simulink model "DeltaWingPlantADRC"  (R2020b)
settings: Solver=VariableStepAuto  StartTime=0.0  StopTime=60  MaxStep=0.01  RelTol=1e-3  EnableMultiTasking=on
values from neighbouring files (symbols this model uses):
  B = [0; 1]    [init.m]    (also in init_adrc.m = [0; theta6; 0])
  Ba = Ta*B    [init_adrc.m]
  beta0 = 0.4    [init_adrc.m]
  betap0 = 0    [init_adrc.m]
  gamma = A - L*C    [init_adrc.m]
  gamma_a = I + Ta*gamma    [init_adrc.m]
  kd = 2*wc + theta20    (= 6.29818530718)    [init_adrc.m]
  kp = wc^2+ theta10    (= 9.85160440109)    [init_adrc.m]
  L = [l1; l2; l3]    [init_adrc.m]
  La = Ta*L    [init_adrc.m]
  Ta = 0.04    [init_adrc.m]    (also in init_miac.m = 0.05)
  Tc = 0.1    [init_adrc.m]    (also in init_miac.m = 0.001; init_mrac.m; init_mraclb.m)
  theta10 = -0.018    [init_adrc.m]
  theta20 = 0.015    [init_adrc.m]
  theta6 = 0.5    [init_adrc.m]
libraries: simulink x2
settings Model: Creator=Melkamu A  LastModifiedBy=Melkamu A
settings DataIOCC: LimitDataPoints=on  SaveFormat=Array  SignalLoggingSaveFormat=ModelDataLogs  ReturnWorkspaceOutputs=off
settings OptimizationCC: InitFltsAndDblsToZero=on  LifeSpan=inf
settings DebuggingCC: SaveWithParameterizedLinksMsg=none  UnderspecifiedInitializationDetection=Classic  MergeDetectMultiDrivingBlocksExec=none  SignalResolutionControl=TryResolveAllWithWarning  SolverPrmCheckMsg=warning  MultiTaskDSMMsg=warning  MultiTaskCondExecSysMsg=none  FcnCallInpInsideContextMsg=warning  SFUnexpectedBacktrackingDiag=warning  SFNoUnconditionalDefaultTransitionDiag=warning  SFExecutionAtInitializationDiag=none  ArithmeticOperatorsInVariantConditions=warning
settings HardwareCC: ProdBitPerPointer=32  ProdBitPerSizeT=32  ProdBitPerPtrDiffT=32  ProdLargestAtomicFloat=None  ProdIntDivRoundTo=Undefined  ProdEndianess=Unspecified  ProdWordSize=32  ProdHWDeviceType=32-bit Generic
settings ModelReferenceCC: PropagateSignalLabelsOutOfModel=off
settings CodeAppCC: StateflowObjectComments=on
settings GRTTargetCC: TargetFcnLib=ansi_tfl_tmw.mat  TargetLangStandard=C89/C90 (ANSI)  CombineOutputUpdateFcns=off  GRTInterface=on
settings ConfigComp: CovMetricSettings=dw  CovSaveCumulativeToWorkspaceVar=on  CovSaveSingleToWorkspaceVar=on

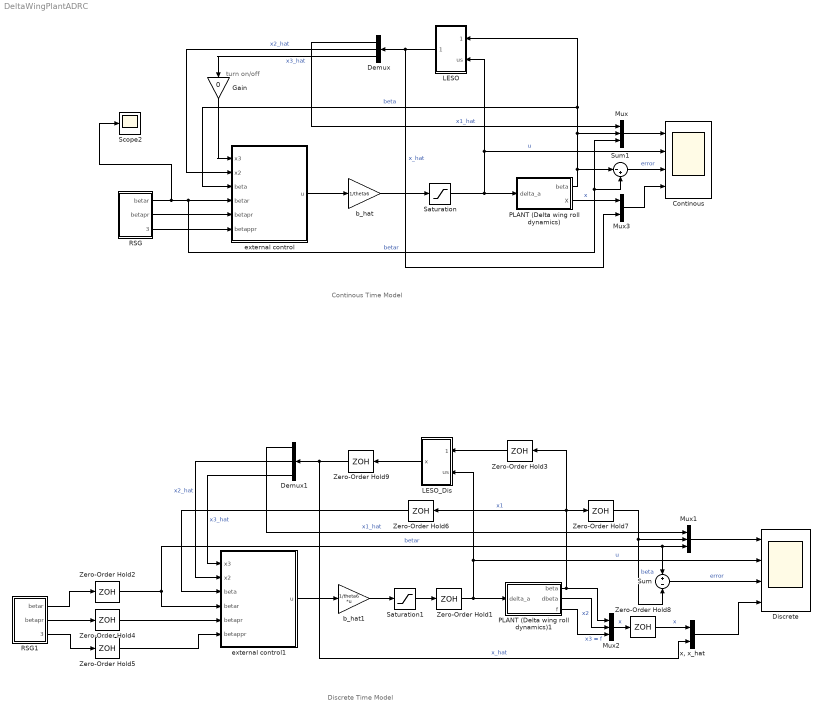
== system DeltaWingPlantADRC ==
  note: turn on/off
  note: Discrete Time Model
  note: Continous Time Model
  Continous : Scope  NumInputPorts=4
  Demux : Demux  Outputs=3
  Demux1 : Demux  Outputs=3
  Discrete : Scope  NumInputPorts=4
  Gain : Gain  Gain=0
  LESO : Subsystem
  LESO_Dis : Subsystem
  Mux : Mux  Inputs=3
  Mux1 : Mux  Inputs=3
  Mux2 : Mux  Inputs=3
  Mux3 : Mux  Inputs=2
  PLANT (Delta wing roll dynamics) : Subsystem
  PLANT (Delta wing roll dynamics)1 : Subsystem
  RSG : Subsystem
  RSG1 : Subsystem
  Saturation : Saturate  UpperLimit=pi  LowerLimit=-pi
  Saturation1 : Saturate  UpperLimit=pi  LowerLimit=-pi
  Scope2 : Scope
  Sum : Sum  Inputs=+-
  Sum1 : Sum  Inputs=|-+
  Zero-Order Hold{1..2,4..9} (8 alike) : ZeroOrderHold  SampleTime=Tc
  Zero-Order Hold3 : ZeroOrderHold  SampleTime=Ta
  b_hat : Gain  Gain=1/theta6
  b_hat1 : Gain  Gain=1/theta6  Multiplication=Matrix(K*u)
  external control : Subsystem
  external control1 : Subsystem
  "x, x_hat" : Mux  Inputs=2
  wires:
  b_hat/1 -> Saturation/1
  PLANT (Delta wing roll dynamics)/1(beta) -> Sum1/1, LESO/1(beta), external control/3(beta), Mux/2  "beta"
  RSG/1(betar) -> Scope2/1, Sum1/2, Mux/3, external control/4(betar)  "betar"
  RSG/2(betapr) -> external control/5(betapr)
  RSG/3(betappr) -> external control/6(betappr)
  external control/1(u) -> b_hat/1
  Demux/3 -> Gain/1  "x3_hat"
  Saturation/1 -> LESO/2(us), Continous/2, PLANT (Delta wing roll dynamics)/1(delta_a)  "u"
  Demux/2 -> external control/2(x2)  "x2_hat"
  Mux/1 -> Continous/1
  Demux/1 -> Mux/1  "x1_hat"
  Demux1/1 -> Mux1/1  "x1_hat"
  Mux1/1 -> Discrete/1
  Demux1/2 -> external control1/2(x2)  "x2_hat"
  b_hat1/1 -> Saturation1/1
  Demux1/3 -> external control1/1(x3)  "x3_hat"
  external control1/1(u) -> b_hat1/1
  RSG1/3(betappr) -> Zero-Order Hold5/1
  RSG1/2(betapr) -> Zero-Order Hold4/1
  RSG1/1(betar) -> Zero-Order Hold2/1
  Zero-Order Hold1/1 -> PLANT (Delta wing roll dynamics)1/1(delta_a), LESO_Dis/2(us), Discrete/2  "u"
  PLANT (Delta wing roll dynamics)1/1(beta) -> Mux2/1, Zero-Order Hold3/1, Zero-Order Hold7/1, Zero-Order Hold6/1  "x1"
  Zero-Order Hold3/1 -> LESO_Dis/1(beta)
  Zero-Order Hold2/1 -> Mux1/3, Sum/1, external control1/4(betar)  "betar"
  Zero-Order Hold5/1 -> external control1/6(betappr)
  Zero-Order Hold4/1 -> external control1/5(betapr)
  Zero-Order Hold6/1 -> external control1/3(beta)
  Saturation1/1 -> Zero-Order Hold1/1
  PLANT (Delta wing roll dynamics)1/3(f) -> Mux2/3  "x3 = f"
  PLANT (Delta wing roll dynamics)1/2(dbeta) -> Mux2/2  "x2"
  "x, x_hat"/1 -> Discrete/4
  Sum/1 -> Discrete/3  "error"
  LESO/1(x_hat) -> Demux/1, Mux3/2  "x_hat"
  PLANT (Delta wing roll dynamics)/2(X) -> Mux3/1  "x"
  Mux3/1 -> Continous/4
  Sum1/1 -> Continous/3  "error"
  LESO_Dis/1(x) -> Zero-Order Hold9/1
  Mux2/1 -> Zero-Order Hold8/1  "x"
  Gain/1 -> external control/1(x3)
  Zero-Order Hold7/1 -> Mux1/2, Sum/2  "beta"
  Zero-Order Hold8/1 -> "x, x_hat"/1  "x"
  Zero-Order Hold9/1 -> "x, x_hat"/2, Demux1/1  "x_hat"

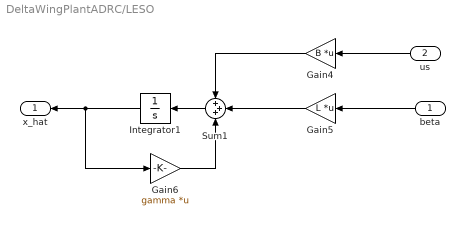
== system DeltaWingPlantADRC/LESO ==
  beta : Inport
  us : Inport  Port=2
  Gain4 : Gain  Gain=B  Multiplication=Matrix(K*u)
  Gain5 : Gain  Gain=L  Multiplication=Matrix(K*u)
  Gain6 : Gain  Gain=gamma  Multiplication=Matrix(K*u)
  Integrator1 : Integrator
  Sum1 : Sum  Inputs=+++
  x_hat : Outport
  wires:
  us/1 -> Gain4/1
  beta/1 -> Gain5/1
  Gain4/1 -> Sum1/1
  Gain5/1 -> Sum1/2
  Gain6/1 -> Sum1/3
  Sum1/1 -> Integrator1/1
  Integrator1/1 -> x_hat/1, Gain6/1

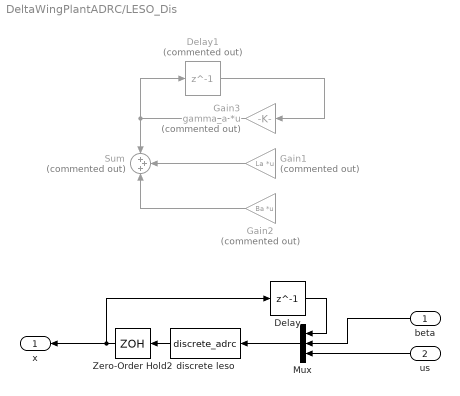
== system DeltaWingPlantADRC/LESO_Dis ==
  beta : Inport
  us : Inport  Port=2
  Delay : Delay  DelayLength=1  SampleTime=Ta
  Delay1 : Delay  Commented=on  DelayLength=1
  Gain1 : Gain  Commented=on  Gain=La  Multiplication=Matrix(K*u)
  Gain2 : Gain  Commented=on  Gain=Ba  Multiplication=Matrix(K*u)
  Gain3 : Gain  Commented=on  Gain=gamma_a  Multiplication=Matrix(K*u)
  Mux : Mux  Inputs=[3 1 1]
  Sum : Sum  Commented=on  Inputs=+++
  Zero-Order Hold2 : ZeroOrderHold  SampleTime=Ta
  "discrete leso " : MATLABFcn  MATLABFcn=discrete_adrc  OutputDimensions=3
  x : Outport
  wires:
  Gain2/1 -> Sum/3
  Gain1/1 -> Sum/2
  Gain3/1 -> Delay1/1, Sum/1
  Mux/1 -> "discrete leso "/1
  "discrete leso "/1 -> Zero-Order Hold2/1
  Zero-Order Hold2/1 -> Delay/1, x/1
  Delay/1 -> Mux/1
  Delay1/1 -> Gain3/1
  beta/1 -> Mux/2
  us/1 -> Mux/3

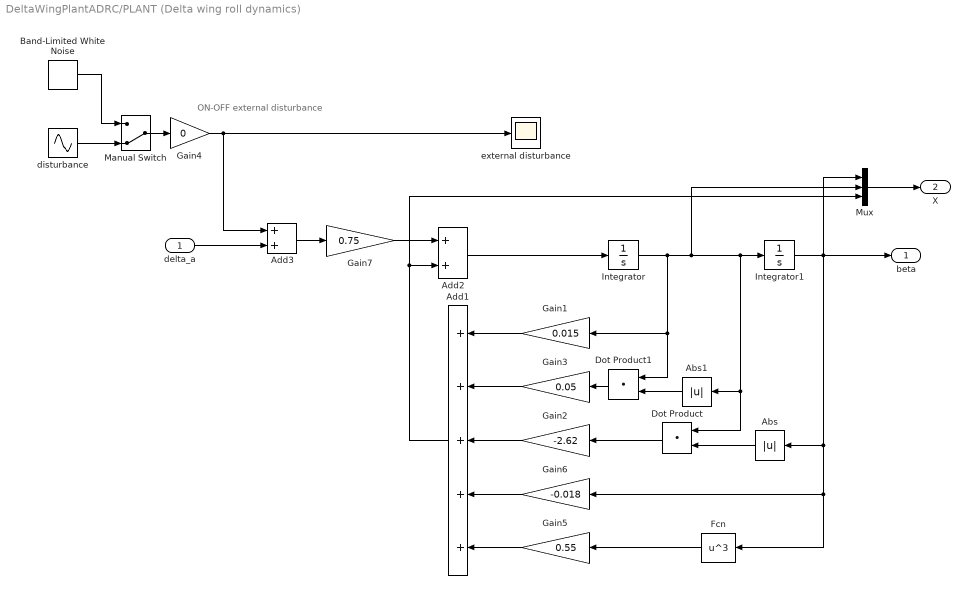
== system DeltaWingPlantADRC/PLANT (Delta wing roll dynamics) ==
  note: ON-OFF external
      | disturbance
  delta_a : Inport
  Abs : Abs
  Abs1 : Abs
  Add1 : Sum  Inputs=+++++
  Add2 : Sum
  Add3 : Sum
  Band-Limited White Noise : simulink/Sources/Band-Limited White Noise  Cov=[0.1*15]  Ts=15  seed=[23341]
  Dot Product : DotProduct  InputSameDT=on  OutDataTypeStr=Inherit: Inherit via internal rule
  Dot Product1 : DotProduct  InputSameDT=on  OutDataTypeStr=Inherit: Inherit via internal rule
  Fcn : Fcn  Expr=u^3
  Gain1 : Gain  Gain=0.015
  Gain2 : Gain  Gain=-2.62
  Gain3 : Gain  Gain=0.05
  Gain4 : Gain  Gain=0
  Gain5 : Gain  Gain=0.55
  Gain6 : Gain  Gain=-0.018
  Gain7 : Gain  Gain=0.75
  Integrator : Integrator  InitialCondition=betap0
  Integrator1 : Integrator  InitialCondition=beta0
  Manual Switch : ManualSwitch  CurrentSetting=0
  Mux : Mux  Inputs=3
  disturbance : Sin  Amplitude=1.5  SampleTime=0
  external disturbance : Scope
  beta : Outport
  X : Outport  Port=2
  wires:
  Integrator/1 -> Dot Product1/1, Gain1/1, Mux/2, Integrator1/1, Dot Product/1, Abs1/1
  Add2/1 -> Integrator/1
  Manual Switch/1 -> Gain4/1
  Band-Limited White Noise/1 -> Manual Switch/1
  disturbance/1 -> Manual Switch/2
  Integrator1/1 -> Mux/1, Gain6/1, Fcn/1, Abs/1, beta/1
  Add1/1 -> Mux/3, Add2/2
  Fcn/1 -> Gain5/1
  Dot Product/1 -> Gain2/1
  Abs/1 -> Dot Product/2
  Abs1/1 -> Dot Product1/2
  Dot Product1/1 -> Gain3/1
  Gain1/1 -> Add1/1
  Gain3/1 -> Add1/2
  Gain2/1 -> Add1/3
  Gain6/1 -> Add1/4
  Gain5/1 -> Add1/5
  Gain4/1 -> external disturbance/1, Add3/1
  Add3/1 -> Gain7/1
  delta_a/1 -> Add3/2
  Gain7/1 -> Add2/1
  Mux/1 -> X/1

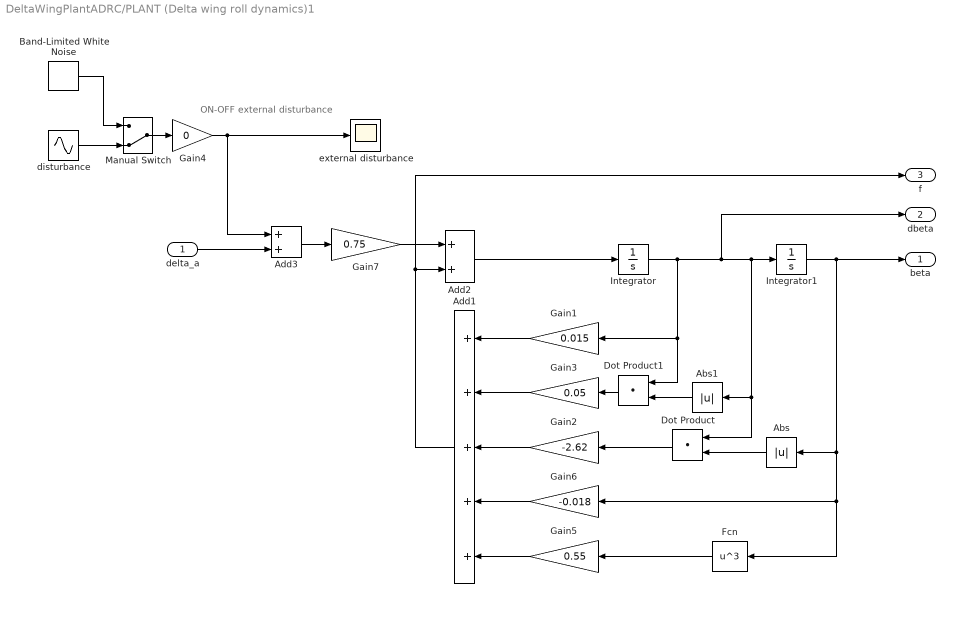
== system DeltaWingPlantADRC/PLANT (Delta wing roll dynamics)1 ==
  note: ON-OFF external
      | disturbance
  delta_a : Inport
  Abs : Abs
  Abs1 : Abs
  Add1 : Sum  Inputs=+++++
  Add2 : Sum
  Add3 : Sum
  Band-Limited White Noise : simulink/Sources/Band-Limited White Noise  Cov=[0.1*15]  Ts=15  seed=[23341]
  Dot Product : DotProduct  InputSameDT=on  OutDataTypeStr=Inherit: Inherit via internal rule
  Dot Product1 : DotProduct  InputSameDT=on  OutDataTypeStr=Inherit: Inherit via internal rule
  Fcn : Fcn  Expr=u^3
  Gain1 : Gain  Gain=0.015
  Gain2 : Gain  Gain=-2.62
  Gain3 : Gain  Gain=0.05
  Gain4 : Gain  Gain=0
  Gain5 : Gain  Gain=0.55
  Gain6 : Gain  Gain=-0.018
  Gain7 : Gain  Gain=0.75
  Integrator : Integrator  InitialCondition=betap0
  Integrator1 : Integrator  InitialCondition=beta0
  Manual Switch : ManualSwitch  CurrentSetting=0
  disturbance : Sin  Amplitude=1.5  SampleTime=0
  external disturbance : Scope
  beta : Outport
  dbeta : Outport  Port=2
  f : Outport  Port=3
  wires:
  Gain7/1 -> Add2/1
  delta_a/1 -> Add3/2
  Add3/1 -> Gain7/1
  Gain4/1 -> Add3/1, external disturbance/1
  Gain5/1 -> Add1/5
  Gain6/1 -> Add1/4
  Gain2/1 -> Add1/3
  Gain3/1 -> Add1/2
  Gain1/1 -> Add1/1
  Dot Product1/1 -> Gain3/1
  Abs1/1 -> Dot Product1/2
  Abs/1 -> Dot Product/2
  Dot Product/1 -> Gain2/1
  Fcn/1 -> Gain5/1
  Add1/1 -> f/1, Add2/2
  Integrator1/1 -> Abs/1, Fcn/1, Gain6/1, beta/1
  disturbance/1 -> Manual Switch/2
  Band-Limited White Noise/1 -> Manual Switch/1
  Manual Switch/1 -> Gain4/1
  Add2/1 -> Integrator/1
  Integrator/1 -> dbeta/1, Abs1/1, Dot Product/1, Integrator1/1, Gain1/1, Dot Product1/1

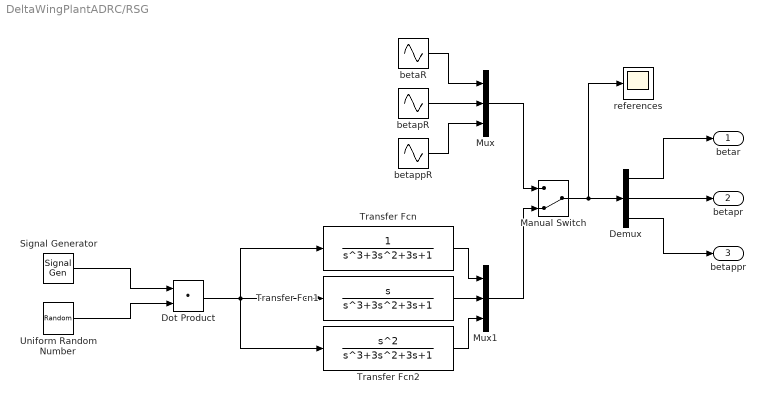
== system DeltaWingPlantADRC/RSG ==
  Demux : Demux  Outputs=3
  Dot Product : DotProduct  InputSameDT=on  OutDataTypeStr=Inherit: Inherit via internal rule
  Manual Switch : ManualSwitch  CurrentSetting=0
  Mux : Mux  Inputs=3
  Mux1 : Mux  Inputs=3
  Signal Generator : SignalGenerator  WaveForm=square  Frequency=0.05
  Transfer Fcn : TransferFcn  Denominator=[1 3 3 1]
  Transfer Fcn1 : TransferFcn  Numerator=[1 0]  Denominator=[1 3 3 1]
  Transfer Fcn2 : TransferFcn  Numerator=[1 0 0]  Denominator=[1 3 3 1]
  Uniform Random Number : UniformRandomNumber  Minimum=-0.8*pi/2  Maximum=0.8*pi/2  SampleTime=10
  betaR : Sin  Frequency=0.5  SampleTime=0
  betapR : Sin  Amplitude=0.5  Frequency=0.5  Phase=pi/2  SampleTime=0
  betappR : Sin  Amplitude=-1*0.5*0.5  Frequency=0.5  SampleTime=0
  references : Scope
  betar : Outport
  betapr : Outport  Port=2
  betappr : Outport  Port=3
  wires:
  betaR/1 -> Mux/1
  betapR/1 -> Mux/2
  betappR/1 -> Mux/3
  Mux/1 -> Manual Switch/1
  Mux1/1 -> Manual Switch/2
  Manual Switch/1 -> Demux/1, references/1
  Demux/2 -> betapr/1
  Demux/1 -> betar/1
  Demux/3 -> betappr/1
  Transfer Fcn/1 -> Mux1/1
  Transfer Fcn1/1 -> Mux1/2
  Transfer Fcn2/1 -> Mux1/3
  Signal Generator/1 -> Dot Product/1
  Uniform Random Number/1 -> Dot Product/2
  Dot Product/1 -> Transfer Fcn2/1, Transfer Fcn/1, Transfer Fcn1/1

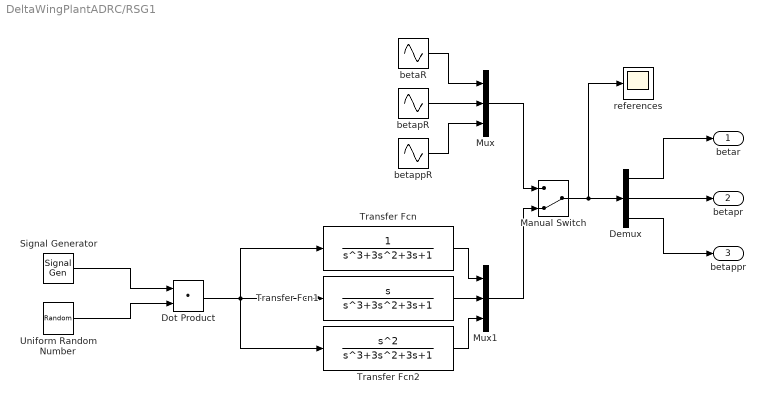
== system DeltaWingPlantADRC/RSG1 ==
  Demux : Demux  Outputs=3
  Dot Product : DotProduct  InputSameDT=on  OutDataTypeStr=Inherit: Inherit via internal rule
  Manual Switch : ManualSwitch  CurrentSetting=0
  Mux : Mux  Inputs=3
  Mux1 : Mux  Inputs=3
  Signal Generator : SignalGenerator  WaveForm=square  Frequency=0.05
  Transfer Fcn : TransferFcn  Denominator=[1 3 3 1]
  Transfer Fcn1 : TransferFcn  Numerator=[1 0]  Denominator=[1 3 3 1]
  Transfer Fcn2 : TransferFcn  Numerator=[1 0 0]  Denominator=[1 3 3 1]
  Uniform Random Number : UniformRandomNumber  Minimum=-0.8*pi/2  Maximum=0.8*pi/2  SampleTime=10
  betaR : Sin  Frequency=0.5  SampleTime=0
  betapR : Sin  Amplitude=0.5  Frequency=0.5  Phase=pi/2  SampleTime=0
  betappR : Sin  Amplitude=-1*0.5*0.5  Frequency=0.5  SampleTime=0
  references : Scope
  betar : Outport
  betapr : Outport  Port=2
  betappr : Outport  Port=3
  wires:
  Dot Product/1 -> Transfer Fcn1/1, Transfer Fcn/1, Transfer Fcn2/1
  Uniform Random Number/1 -> Dot Product/2
  Signal Generator/1 -> Dot Product/1
  Transfer Fcn2/1 -> Mux1/3
  Transfer Fcn1/1 -> Mux1/2
  Transfer Fcn/1 -> Mux1/1
  Demux/3 -> betappr/1
  Demux/1 -> betar/1
  Demux/2 -> betapr/1
  Manual Switch/1 -> references/1, Demux/1
  Mux1/1 -> Manual Switch/2
  Mux/1 -> Manual Switch/1
  betappR/1 -> Mux/3
  betapR/1 -> Mux/2
  betaR/1 -> Mux/1

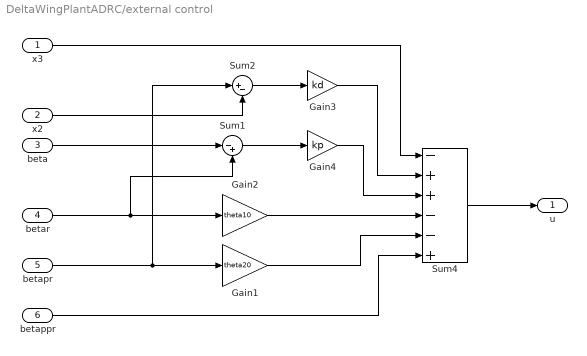
== system DeltaWingPlantADRC/external control ==
  x3 : Inport
  x2 : Inport  Port=2
  beta : Inport  Port=3
  betar : Inport  Port=4
  betapr : Inport  Port=5
  betappr : Inport  Port=6
  Gain1 : Gain  Gain=theta20
  Gain2 : Gain  Gain=theta10
  Gain3 : Gain  Gain=kd
  Gain4 : Gain  Gain=kp
  Sum1 : Sum  Inputs=|-+
  Sum2 : Sum  Inputs=|+-
  Sum4 : Sum  Inputs=-++--+
  u : Outport
  wires:
  x3/1 -> Sum4/1
  beta/1 -> Sum1/1
  betapr/1 -> Gain1/1, Sum2/1
  x2/1 -> Sum2/2
  betar/1 -> Sum1/2, Gain2/1
  Gain3/1 -> Sum4/2
  Sum2/1 -> Gain3/1
  betappr/1 -> Sum4/6
  Sum1/1 -> Gain4/1
  Gain2/1 -> Sum4/4
  Gain4/1 -> Sum4/3
  Sum4/1 -> u/1
  Gain1/1 -> Sum4/5

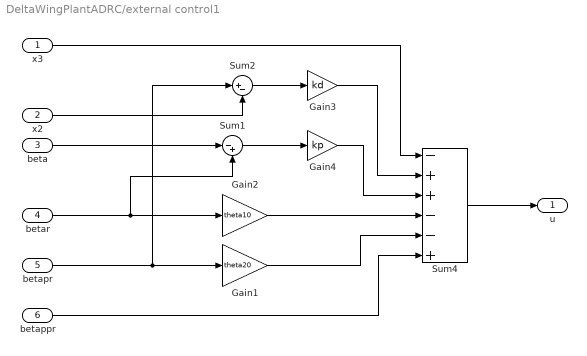
== system DeltaWingPlantADRC/external control1 ==
  x3 : Inport
  x2 : Inport  Port=2
  beta : Inport  Port=3
  betar : Inport  Port=4
  betapr : Inport  Port=5
  betappr : Inport  Port=6
  Gain1 : Gain  Gain=theta20
  Gain2 : Gain  Gain=theta10
  Gain3 : Gain  Gain=kd
  Gain4 : Gain  Gain=kp
  Sum1 : Sum  Inputs=|-+
  Sum2 : Sum  Inputs=|+-
  Sum4 : Sum  Inputs=-++--+
  u : Outport
  wires:
  Gain1/1 -> Sum4/5
  Sum4/1 -> u/1
  Gain4/1 -> Sum4/3
  Gain2/1 -> Sum4/4
  Sum1/1 -> Gain4/1
  Sum2/1 -> Gain3/1
  Gain3/1 -> Sum4/2
  beta/1 -> Sum1/1
  x3/1 -> Sum4/1
  betar/1 -> Gain2/1, Sum1/2
  betapr/1 -> Sum2/1, Gain1/1
  betappr/1 -> Sum4/6
  x2/1 -> Sum2/2
